simulink model "Two_Zone_MVDC_Ideal_ACDC"  (R2020b)
settings: Solver=FixedStepDiscrete  StartTime=0.0  StopTime=50  FixedStep=TsELEC  RelTol=1e-3  EnableMultiTasking=on
InitFcn:
  | TsELEC = 5e-4;
  | Ts = 5e-4;
undefined symbols (not defined in the file): DiscIntNeverNeededParam, droop1, droop2, GABDA, GABDB, GBBDA, GBBDB, GPMMA, GPPMB, GPPMC, SADA, SADB, SADC, SADD, SBDA, SBDB, SBDC, SCDA, SCDB, SCDC, SCDD, SDDA, SDDB, SDDC, SDDD, SDDE
libraries: fl_lib x66, nesl_utility x49, ee_lib x30, simulink x1
(part 1 of 2)
CloseFcn:
  | load initParams
settings Model: SimulationMode=accelerator  Creator=gdudgeon  LastModifiedBy=gdudgeon
settings SolverCC: ConcurrentTasks=on  AutoInsertRateTranBlk=on
settings DataIOCC: SaveFormat=StructureWithTime  SaveOutput=off  DSMLogging=off  SaveTime=off  ReturnWorkspaceOutputs=off
settings OptimizationCC: BlockReduction=off  OptimizeBlockIOStorage=off  BufferReuse=off  GlobalBufferReuse=off  ExpressionFolding=off  LocalBlockOutputs=off  OptimizeDataStoreBuffers=off  BusAssignmentInplaceUpdate=off
settings ModelReferenceCC: ModelReferenceNumInstancesAllowed=Single  ModelReferenceMinAlgLoopOccurrences=on
settings SFSimCC: CustomCodeUndefinedFunction=UseInterfaceOnly
settings RTWCC: TLCOptions=-axPCMaxOverloads=3000  RTWCompilerOptimization=on
settings GRTTargetCC: TargetLangStandard=C89/C90 (ANSI)

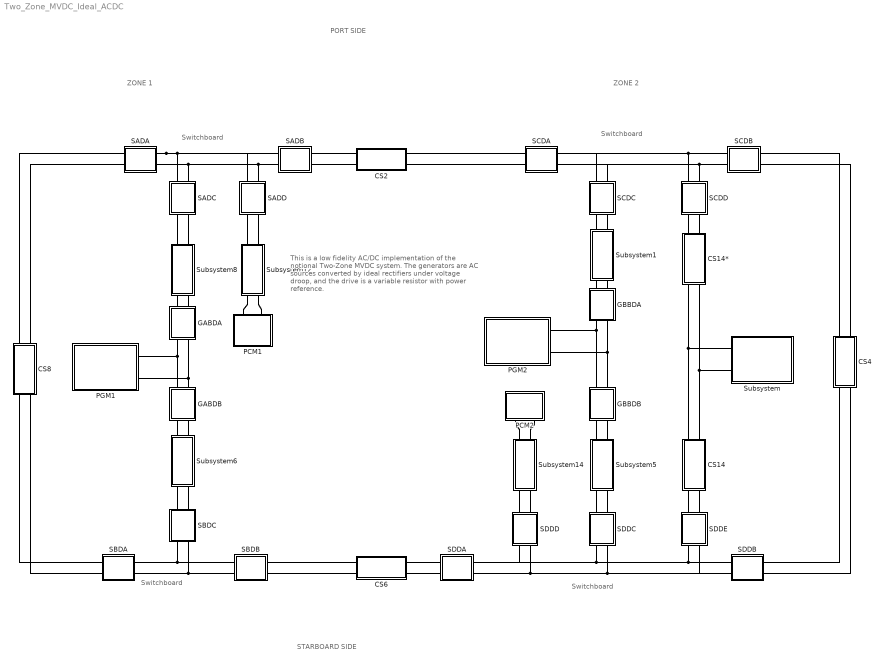
== system Two_Zone_MVDC_Ideal_ACDC ==
  note: This is a low fidelity
      | AC/DC implementation of the notional
      | Two-Zone MVDC system.
      | The generators are AC sources converted by ideal rectifiers under voltage droop, and the drive is a variable resistor with power reference.
  note: PORT SIDE
  note: Switchboard
  note: ZONE 1
  note: ZONE 2
  note: Switchboard
  note: Switchboard
  note: Switchboard
  note: STARBOARD SIDE
  CS14 : Subsystem
      mask Display: disp('CS14')
  CS14* : Subsystem
      mask Display: disp('CS14*')
  CS2 : Subsystem
      mask Display: disp('CS2')
  CS4 : Subsystem
      mask Display: disp('CS4')
  CS6 : Subsystem
      mask Display: disp('CS6')
  CS8 : Subsystem
      mask Display: disp('CS8')
  GABDA : Subsystem  mask{status=GABDA}
      mask prompts: status "Initial Status"
      mask init:
      | if ~status
      |     
      |     set(gcbh,'BackgroundColor','green')
      |     
      | elseif status
      |     
      |     set(gcbh,'BackgroundColor','red')
      |     
      | end
  GABDB : Subsystem  mask{status=GABDB}
      mask prompts: status "Initial Status"
      mask init:
      | if ~status
      |     
      |     set(gcbh,'BackgroundColor','green')
      |     
      | elseif status
      |     
      |     set(gcbh,'BackgroundColor','red')
      |     
      | end
  GBBDA : Subsystem  mask{status=GBBDA}
      mask prompts: status "Initial Status"
      mask init:
      | if ~status
      |     
      |     set(gcbh,'BackgroundColor','green')
      |     
      | elseif status
      |     
      |     set(gcbh,'BackgroundColor','red')
      |     
      | end
  GBBDB : Subsystem  mask{status=GBBDB}
      mask prompts: status "Initial Status"
      mask init:
      | if ~status
      |     
      |     set(gcbh,'BackgroundColor','green')
      |     
      | elseif status
      |     
      |     set(gcbh,'BackgroundColor','red')
      |     
      | end
  PCM1 : Subsystem
      mask Display: disp('PCM1')
  PCM2 : Subsystem
      mask Display: disp('PCM2')
  PGM1 : Subsystem
      mask Display: disp('PGM1')
  PGM2 : Subsystem
      mask Display: disp('PGM2')
  SADA : Subsystem  mask{status=SADA}
      mask prompts: status "Initial Status"
      mask init:
      | if ~status
      |     
      |     set(gcbh,'BackgroundColor','green')
      |     
      | elseif status
      |     
      |     set(gcbh,'BackgroundColor','red')
      |     
      | end
  SADB : Subsystem  mask{status=SADB}
      mask prompts: status "Initial Status"
      mask init:
      | if ~status
      |     
      |     set(gcbh,'BackgroundColor','green')
      |     
      | elseif status
      |     
      |     set(gcbh,'BackgroundColor','red')
      |     
      | end
  SADC : Subsystem  mask{status=SADC}
      mask prompts: status "Initial Status"
      mask init:
      | if ~status
      |     
      |     set(gcbh,'BackgroundColor','green')
      |     
      | elseif status
      |     
      |     set(gcbh,'BackgroundColor','red')
      |     
      | end
  SADD : Subsystem  mask{status=SADD}
      mask prompts: status "Initial Status"
      mask init:
      | if ~status
      |     
      |     set(gcbh,'BackgroundColor','green')
      |     
      | elseif status
      |     
      |     set(gcbh,'BackgroundColor','red')
      |     
      | end
  SBDA : Subsystem  mask{status=SBDA}
      mask prompts: status "Initial Status"
      mask init:
      | if ~status
      |     
      |     set(gcbh,'BackgroundColor','green')
      |     
      | elseif status
      |     
      |     set(gcbh,'BackgroundColor','red')
      |     
      | end
  SBDB : Subsystem  mask{status=SBDB}
      mask prompts: status "Initial Status"
      mask init:
      | if ~status
      |     
      |     set(gcbh,'BackgroundColor','green')
      |     
      | elseif status
      |     
      |     set(gcbh,'BackgroundColor','red')
      |     
      | end
  SBDC : Subsystem  mask{status=SBDC}
      mask prompts: status "Initial Status"
      mask init:
      | if ~status
      |     
      |     set(gcbh,'BackgroundColor','green')
      |     
      | elseif status
      |     
      |     set(gcbh,'BackgroundColor','red')
      |     
      | end
  SCDA : Subsystem  mask{status=SCDA}
      mask prompts: status "Initial Status"
      mask init:
      | if ~status
      |     
      |     set(gcbh,'BackgroundColor','green')
      |     
      | elseif status
      |     
      |     set(gcbh,'BackgroundColor','red')
      |     
      | end
  SCDB : Subsystem  mask{status=SCDB}
      mask prompts: status "Initial Status"
      mask init:
      | if ~status
      |     
      |     set(gcbh,'BackgroundColor','green')
      |     
      | elseif status
      |     
      |     set(gcbh,'BackgroundColor','red')
      |     
      | end
  SCDC : Subsystem  mask{status=SCDC}
      mask prompts: status "Initial Status"
      mask init:
      | if ~status
      |     
      |     set(gcbh,'BackgroundColor','green')
      |     
      | elseif status
      |     
      |     set(gcbh,'BackgroundColor','red')
      |     
      | end
  SCDD : Subsystem  mask{status=SCDD}
      mask prompts: status "Initial Status"
      mask init:
      | if ~status
      |     
      |     set(gcbh,'BackgroundColor','green')
      |     
      | elseif status
      |     
      |     set(gcbh,'BackgroundColor','red')
      |     
      | end
  SDDA : Subsystem  mask{status=SDDA}
      mask prompts: status "Initial Status"
      mask init:
      | if ~status
      |     
      |     set(gcbh,'BackgroundColor','green')
      |     
      | elseif status
      |     
      |     set(gcbh,'BackgroundColor','red')
      |     
      | end
  SDDB : Subsystem  mask{status=SDDB}
      mask prompts: status "Initial Status"
      mask init:
      | if ~status
      |     
      |     set(gcbh,'BackgroundColor','green')
      |     
      | elseif status
      |     
      |     set(gcbh,'BackgroundColor','red')
      |     
      | end
  SDDC : Subsystem  mask{status=SDDC}
      mask prompts: status "Initial Status"
      mask init:
      | if ~status
      |     
      |     set(gcbh,'BackgroundColor','green')
      |     
      | elseif status
      |     
      |     set(gcbh,'BackgroundColor','red')
      |     
      | end
  SDDD : Subsystem  mask{status=SDDD}
      mask prompts: status "Initial Status"
      mask init:
      | if ~status
      |     
      |     set(gcbh,'BackgroundColor','green')
      |     
      | elseif status
      |     
      |     set(gcbh,'BackgroundColor','red')
      |     
      | end
  SDDE : Subsystem  mask{status=SDDE}
      mask prompts: status "Initial Status"
      mask init:
      | if ~status
      |     
      |     set(gcbh,'BackgroundColor','green')
      |     
      | elseif status
      |     
      |     set(gcbh,'BackgroundColor','red')
      |     
      | end
  Subsystem : Subsystem
      mask Display: disp('PMM')
  Subsystem1 : Subsystem
      mask Display: disp('CS11*')
  Subsystem12 : Subsystem
      mask Display: disp('CS21')
  Subsystem14 : Subsystem
      mask Display: disp('CS22')
  Subsystem5 : Subsystem
      mask Display: disp('CS11')
  Subsystem6 : Subsystem
      mask Display: disp('CS9*')
  Subsystem8 : Subsystem
      mask Display: disp('CS9')
  connections:
  SADA/RConn2 -- SADC/LConn2 -- SADD/LConn2 -- SADB/LConn2
  SBDC/RConn2 -- SBDB/LConn2 -- SBDA/RConn2
  PGM1/RConn2 -- GABDB/LConn2 -- GABDA/RConn2
  PGM1/RConn1 -- GABDB/LConn1 -- GABDA/RConn1
  SADA/RConn1 -- SADD/LConn1 -- SADB/LConn1 -- SADC/LConn1
  SBDC/RConn1 -- SBDB/LConn1 -- SBDA/RConn1
  SCDA/LConn2 -- CS2/LConn2
  SADB/RConn1 -- CS2/RConn1
  Subsystem12/LConn1 -- SADD/RConn1
  SBDA/LConn2 -- CS8/RConn2
  SBDC/LConn1 -- Subsystem6/RConn1
  Subsystem12/RConn1 -- PCM1/LConn1
  SBDB/RConn1 -- CS6/RConn1
  SBDC/LConn2 -- Subsystem6/RConn2
  CS8/LConn1 -- SADA/LConn1
  Subsystem12/RConn2 -- PCM1/LConn2
  Subsystem12/LConn2 -- SADD/RConn2
  SADC/RConn1 -- Subsystem8/LConn1
  SBDB/RConn2 -- CS6/RConn2
  SADB/RConn2 -- CS2/RConn2
  CS8/LConn2 -- SADA/LConn2
  SBDA/LConn1 -- CS8/RConn1
  SADC/RConn2 -- Subsystem8/LConn2
  GBBDA/RConn1 -- GBBDB/LConn1 -- PGM2/RConn1
  SDDC/RConn2 -- SDDB/LConn2 -- SDDE/RConn2 -- SDDA/RConn2 -- SDDD/RConn2
  SCDC/LConn2 -- SCDA/RConn2 -- SCDD/LConn2 -- SCDB/LConn2
  SDDC/RConn1 -- SDDA/RConn1 -- SDDD/RConn1 -- SDDB/LConn1 -- SDDE/RConn1
  SCDC/LConn1 -- SCDA/RConn1 -- SCDD/LConn1 -- SCDB/LConn1
  GBBDA/RConn2 -- GBBDB/LConn2 -- PGM2/RConn2
  SCDC/RConn2 -- Subsystem1/LConn2
  SCDB/RConn1 -- CS4/LConn1
  SDDB/RConn1 -- CS4/RConn1
  SDDC/LConn2 -- Subsystem5/RConn2
  SDDB/RConn2 -- CS4/RConn2
  SCDB/RConn2 -- CS4/LConn2
  SDDC/LConn1 -- Subsystem5/RConn1
  SCDC/RConn1 -- Subsystem1/LConn1
  CS2/LConn1 -- SCDA/LConn1
  CS6/LConn1 -- SDDA/LConn1
  CS6/LConn2 -- SDDA/LConn2
  GBBDA/LConn1 -- Subsystem1/RConn1
  GBBDA/LConn2 -- Subsystem1/RConn2
  GBBDB/RConn1 -- Subsystem5/LConn1
  GBBDB/RConn2 -- Subsystem5/LConn2
  GABDA/LConn1 -- Subsystem8/RConn1
  GABDA/LConn2 -- Subsystem8/RConn2
  GABDB/RConn1 -- Subsystem6/LConn1
  GABDB/RConn2 -- Subsystem6/LConn2
  Subsystem14/LConn1 -- PCM2/LConn1
  Subsystem14/LConn2 -- PCM2/LConn2
  Subsystem14/RConn1 -- SDDD/LConn1
  Subsystem14/RConn2 -- SDDD/LConn2
  CS14*/LConn2 -- SCDD/RConn2
  CS14*/LConn1 -- SCDD/RConn1
  CS14/RConn1 -- SDDE/LConn1
  CS14/RConn2 -- SDDE/LConn2
  CS14/LConn1 -- Subsystem/LConn1 -- CS14*/RConn1
  CS14*/RConn2 -- Subsystem/LConn2 -- CS14/LConn2

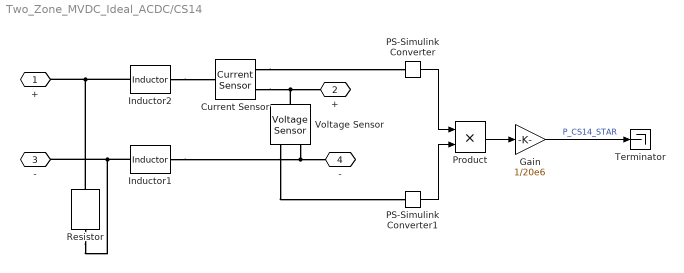
== system Two_Zone_MVDC_Ideal_ACDC/CS14 ==
  Current Sensor : fl_lib/Electrical/Electrical Sensors/Current Sensor
  Gain : Gain  Gain=1/20e6
  Inductor1 : fl_lib/Electrical/Electrical Elements/Inductor  l=5.32e-6 H  r=0.32e-3 Ohm  g=0 1/Ohm  i_specify=off  i_priority=None  i=0 A  i_nominal_specify=off  i_nominal_unit=A  i_nominal_value=1  v_specify=off  v_priority=None  v=0 V  v_nominal_specify=off  v_nominal_unit=V  v_nominal_value=1  i_L_specify=off  i_L_priority=High  i_L=0 A  i_L_nominal_specify=off  i_L_nominal_unit=A  i_L_nominal_value=1
  Inductor2 : fl_lib/Electrical/Electrical Elements/Inductor  l=5.32e-6 H  r=0.32e-3 Ohm  g=0 1/Ohm  i_specify=off  i_priority=None  i=0 A  i_nominal_specify=off  i_nominal_unit=A  i_nominal_value=1  v_specify=off  v_priority=None  v=0 V  v_nominal_specify=off  v_nominal_unit=V  v_nominal_value=1  i_L_specify=off  i_L_priority=High  i_L=0 A  i_L_nominal_specify=off  i_L_nominal_unit=A  i_L_nominal_value=1
  PS-Simulink Converter : nesl_utility/PS-Simulink Converter  PhysicalDomain=network_engine_domain  SubClassName=ps_output  LeftPortType=input  RightPortType=output  PseudoPeriodic=off  Frequencies=[]  Unit=inherit  AffineConversion=off
  PS-Simulink Converter1 : nesl_utility/PS-Simulink Converter  PhysicalDomain=network_engine_domain  SubClassName=ps_output  LeftPortType=input  RightPortType=output  PseudoPeriodic=off  Frequencies=[]  Unit=inherit  AffineConversion=off
  Product : Product
  Resistor : fl_lib/Electrical/Electrical Elements/Resistor  R=1e4 Ohm  i_specify=off  i_priority=None  i=0 A  i_nominal_specify=off  i_nominal_unit=A  i_nominal_value=1  v_specify=off  v_priority=None  v=0 V  v_nominal_specify=off  v_nominal_unit=V  v_nominal_value=1
  Terminator : Terminator
  Voltage Sensor : fl_lib/Electrical/Electrical Sensors/Voltage Sensor
  "+ " : PMIOPort  Side=Left
  + : PMIOPort  Port=2  Side=Right
  - : PMIOPort  Port=3  Side=Left
  "- " : PMIOPort  Port=4  Side=Right
  wires:
  PS-Simulink Converter/1 -> Product/1
  PS-Simulink Converter1/1 -> Product/2
  Product/1 -> Gain/1
  Gain/1 -> Terminator/1  "P_CS14_STAR"
  connections:
  Inductor1/LConn1 -- Resistor/RConn1 -- -/RConn1
  Inductor2/LConn1 -- Resistor/LConn1 -- "+ "/RConn1
  Inductor1/RConn1 -- Voltage Sensor/RConn2 -- "- "/RConn1
  Inductor2/RConn1 -- Current Sensor/LConn1
  Current Sensor/RConn2 -- Voltage Sensor/LConn1 -- +/RConn1
  Current Sensor/RConn1 -- PS-Simulink Converter/LConn1
  Voltage Sensor/RConn1 -- PS-Simulink Converter1/LConn1

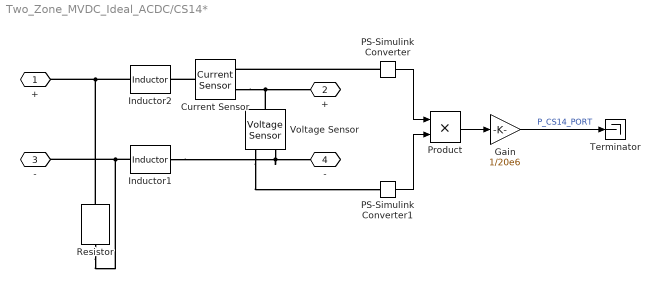
== system Two_Zone_MVDC_Ideal_ACDC/CS14* ==
  Current Sensor : fl_lib/Electrical/Electrical Sensors/Current Sensor
  Gain : Gain  Gain=1/20e6
  Inductor1 : fl_lib/Electrical/Electrical Elements/Inductor  l=5.32e-6 H  r=0.32e-3 Ohm  g=0 1/Ohm  i_specify=off  i_priority=None  i=0 A  i_nominal_specify=off  i_nominal_unit=A  i_nominal_value=1  v_specify=off  v_priority=None  v=0 V  v_nominal_specify=off  v_nominal_unit=V  v_nominal_value=1  i_L_specify=off  i_L_priority=High  i_L=0 A  i_L_nominal_specify=off  i_L_nominal_unit=A  i_L_nominal_value=1
  Inductor2 : fl_lib/Electrical/Electrical Elements/Inductor  l=5.32e-6 H  r=0.32e-3 Ohm  g=0 1/Ohm  i_specify=off  i_priority=None  i=0 A  i_nominal_specify=off  i_nominal_unit=A  i_nominal_value=1  v_specify=off  v_priority=None  v=0 V  v_nominal_specify=off  v_nominal_unit=V  v_nominal_value=1  i_L_specify=off  i_L_priority=High  i_L=0 A  i_L_nominal_specify=off  i_L_nominal_unit=A  i_L_nominal_value=1
  PS-Simulink Converter : nesl_utility/PS-Simulink Converter  PhysicalDomain=network_engine_domain  SubClassName=ps_output  LeftPortType=input  RightPortType=output  PseudoPeriodic=off  Frequencies=[]  Unit=inherit  AffineConversion=off
  PS-Simulink Converter1 : nesl_utility/PS-Simulink Converter  PhysicalDomain=network_engine_domain  SubClassName=ps_output  LeftPortType=input  RightPortType=output  PseudoPeriodic=off  Frequencies=[]  Unit=inherit  AffineConversion=off
  Product : Product
  Resistor : fl_lib/Electrical/Electrical Elements/Resistor  R=1e4 Ohm  i_specify=off  i_priority=None  i=0 A  i_nominal_specify=off  i_nominal_unit=A  i_nominal_value=1  v_specify=off  v_priority=None  v=0 V  v_nominal_specify=off  v_nominal_unit=V  v_nominal_value=1
  Terminator : Terminator
  Voltage Sensor : fl_lib/Electrical/Electrical Sensors/Voltage Sensor
  "+ " : PMIOPort  Side=Left
  + : PMIOPort  Port=2  Side=Right
  - : PMIOPort  Port=3  Side=Left
  "- " : PMIOPort  Port=4  Side=Right
  wires:
  PS-Simulink Converter/1 -> Product/1
  PS-Simulink Converter1/1 -> Product/2
  Product/1 -> Gain/1
  Gain/1 -> Terminator/1  "P_CS14_PORT"
  connections:
  Inductor1/RConn1 -- Voltage Sensor/RConn2 -- "- "/RConn1
  Inductor2/LConn1 -- Resistor/LConn1 -- "+ "/RConn1
  Inductor1/LConn1 -- Resistor/RConn1 -- -/RConn1
  Current Sensor/LConn1 -- Inductor2/RConn1
  Current Sensor/RConn2 -- Voltage Sensor/LConn1 -- +/RConn1
  PS-Simulink Converter/LConn1 -- Current Sensor/RConn1
  Voltage Sensor/RConn1 -- PS-Simulink Converter1/LConn1

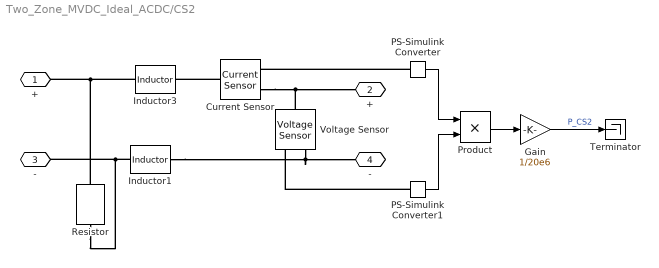
== system Two_Zone_MVDC_Ideal_ACDC/CS2 ==
  Current Sensor : fl_lib/Electrical/Electrical Sensors/Current Sensor
  Gain : Gain  Gain=1/20e6
  Inductor1 : fl_lib/Electrical/Electrical Elements/Inductor  l=3.47e-6 H  r=0.21e-3 Ohm  g=0 1/Ohm  i_specify=off  i_priority=None  i=0 A  i_nominal_specify=off  i_nominal_unit=A  i_nominal_value=1  v_specify=off  v_priority=None  v=0 V  v_nominal_specify=off  v_nominal_unit=V  v_nominal_value=1  i_L_specify=off  i_L_priority=High  i_L=0 A  i_L_nominal_specify=off  i_L_nominal_unit=A  i_L_nominal_value=1
  Inductor3 : fl_lib/Electrical/Electrical Elements/Inductor  l=3.47e-6 H  r=0.21e-3 Ohm  g=0 1/Ohm  i_specify=off  i_priority=None  i=0 A  i_nominal_specify=off  i_nominal_unit=A  i_nominal_value=1  v_specify=off  v_priority=None  v=0 V  v_nominal_specify=off  v_nominal_unit=V  v_nominal_value=1  i_L_specify=off  i_L_priority=High  i_L=0 A  i_L_nominal_specify=off  i_L_nominal_unit=A  i_L_nominal_value=1
  PS-Simulink Converter : nesl_utility/PS-Simulink Converter  PhysicalDomain=network_engine_domain  SubClassName=ps_output  LeftPortType=input  RightPortType=output  PseudoPeriodic=off  Frequencies=[]  Unit=inherit  AffineConversion=off
  PS-Simulink Converter1 : nesl_utility/PS-Simulink Converter  PhysicalDomain=network_engine_domain  SubClassName=ps_output  LeftPortType=input  RightPortType=output  PseudoPeriodic=off  Frequencies=[]  Unit=inherit  AffineConversion=off
  Product : Product
  Resistor : fl_lib/Electrical/Electrical Elements/Resistor  R=1e4 Ohm  i_specify=off  i_priority=None  i=0 A  i_nominal_specify=off  i_nominal_unit=A  i_nominal_value=1  v_specify=off  v_priority=None  v=0 V  v_nominal_specify=off  v_nominal_unit=V  v_nominal_value=1
  Terminator : Terminator
  Voltage Sensor : fl_lib/Electrical/Electrical Sensors/Voltage Sensor
  "+ " : PMIOPort  Side=Left
  + : PMIOPort  Port=2  Side=Right
  - : PMIOPort  Port=3  Side=Left
  "- " : PMIOPort  Port=4  Side=Right
  wires:
  PS-Simulink Converter/1 -> Product/1
  PS-Simulink Converter1/1 -> Product/2
  Product/1 -> Gain/1
  Gain/1 -> Terminator/1  "P_CS2"
  connections:
  Inductor3/LConn1 -- Resistor/LConn1 -- "+ "/RConn1
  Inductor1/LConn1 -- Resistor/RConn1 -- -/RConn1
  Inductor1/RConn1 -- Voltage Sensor/RConn2 -- "- "/RConn1
  Current Sensor/LConn1 -- Inductor3/RConn1
  Current Sensor/RConn2 -- Voltage Sensor/LConn1 -- +/RConn1
  PS-Simulink Converter/LConn1 -- Current Sensor/RConn1
  PS-Simulink Converter1/LConn1 -- Voltage Sensor/RConn1

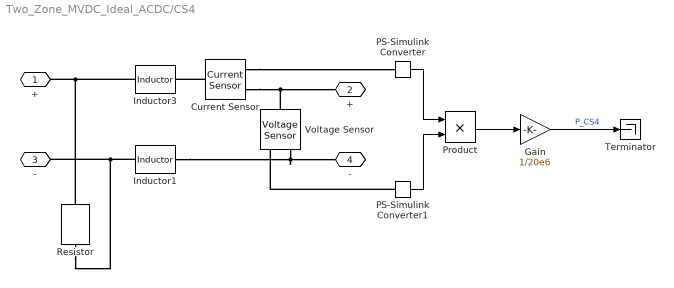
== system Two_Zone_MVDC_Ideal_ACDC/CS4 ==
  Current Sensor : fl_lib/Electrical/Electrical Sensors/Current Sensor
  Gain : Gain  Gain=1/20e6
  Inductor1 : fl_lib/Electrical/Electrical Elements/Inductor  l=5e-6 H  r=0.2e-3 Ohm  g=0 1/Ohm  i_specify=off  i_priority=None  i=0 A  i_nominal_specify=off  i_nominal_unit=A  i_nominal_value=1  v_specify=off  v_priority=None  v=0 V  v_nominal_specify=off  v_nominal_unit=V  v_nominal_value=1  i_L_specify=off  i_L_priority=High  i_L=0 A  i_L_nominal_specify=off  i_L_nominal_unit=A  i_L_nominal_value=1
  Inductor3 : fl_lib/Electrical/Electrical Elements/Inductor  l=5e-6 H  r=0.2e-3 Ohm  g=0 1/Ohm  i_specify=off  i_priority=None  i=0 A  i_nominal_specify=off  i_nominal_unit=A  i_nominal_value=1  v_specify=off  v_priority=None  v=0 V  v_nominal_specify=off  v_nominal_unit=V  v_nominal_value=1  i_L_specify=off  i_L_priority=High  i_L=0 A  i_L_nominal_specify=off  i_L_nominal_unit=A  i_L_nominal_value=1
  PS-Simulink Converter : nesl_utility/PS-Simulink Converter  PhysicalDomain=network_engine_domain  SubClassName=ps_output  LeftPortType=input  RightPortType=output  PseudoPeriodic=off  Frequencies=[]  Unit=inherit  AffineConversion=off
  PS-Simulink Converter1 : nesl_utility/PS-Simulink Converter  PhysicalDomain=network_engine_domain  SubClassName=ps_output  LeftPortType=input  RightPortType=output  PseudoPeriodic=off  Frequencies=[]  Unit=inherit  AffineConversion=off
  Product : Product
  Resistor : fl_lib/Electrical/Electrical Elements/Resistor  R=1e4 Ohm  i_specify=off  i_priority=None  i=0 A  i_nominal_specify=off  i_nominal_unit=A  i_nominal_value=1  v_specify=off  v_priority=None  v=0 V  v_nominal_specify=off  v_nominal_unit=V  v_nominal_value=1
  Terminator : Terminator
  Voltage Sensor : fl_lib/Electrical/Electrical Sensors/Voltage Sensor
  "+ " : PMIOPort  Side=Left
  + : PMIOPort  Port=2  Side=Right
  - : PMIOPort  Port=3  Side=Left
  "- " : PMIOPort  Port=4  Side=Right
  wires:
  Product/1 -> Gain/1
  PS-Simulink Converter/1 -> Product/1
  PS-Simulink Converter1/1 -> Product/2
  Gain/1 -> Terminator/1  "P_CS4"
  connections:
  Inductor3/LConn1 -- Resistor/LConn1 -- "+ "/RConn1
  Inductor1/LConn1 -- Resistor/RConn1 -- -/RConn1
  Current Sensor/LConn1 -- Inductor3/RConn1
  Current Sensor/RConn2 -- Voltage Sensor/LConn1 -- +/RConn1
  Inductor1/RConn1 -- Voltage Sensor/RConn2 -- "- "/RConn1
  Current Sensor/RConn1 -- PS-Simulink Converter/LConn1
  PS-Simulink Converter1/LConn1 -- Voltage Sensor/RConn1

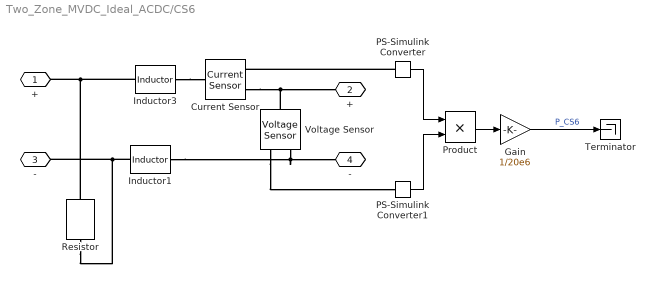
== system Two_Zone_MVDC_Ideal_ACDC/CS6 ==
  Current Sensor : fl_lib/Electrical/Electrical Sensors/Current Sensor
  Gain : Gain  Gain=1/20e6
  Inductor1 : fl_lib/Electrical/Electrical Elements/Inductor  l=3.47e-6 H  r=0.21e-3 Ohm  g=0 1/Ohm  i_specify=off  i_priority=None  i=0 A  i_nominal_specify=off  i_nominal_unit=A  i_nominal_value=1  v_specify=off  v_priority=None  v=0 V  v_nominal_specify=off  v_nominal_unit=V  v_nominal_value=1  i_L_specify=off  i_L_priority=High  i_L=0 A  i_L_nominal_specify=off  i_L_nominal_unit=A  i_L_nominal_value=1
  Inductor3 : fl_lib/Electrical/Electrical Elements/Inductor  l=3.47e-6 H  r=0.21e-3 Ohm  g=0 1/Ohm  i_specify=off  i_priority=None  i=0 A  i_nominal_specify=off  i_nominal_unit=A  i_nominal_value=1  v_specify=off  v_priority=None  v=0 V  v_nominal_specify=off  v_nominal_unit=V  v_nominal_value=1  i_L_specify=off  i_L_priority=High  i_L=0 A  i_L_nominal_specify=off  i_L_nominal_unit=A  i_L_nominal_value=1
  PS-Simulink Converter : nesl_utility/PS-Simulink Converter  PhysicalDomain=network_engine_domain  SubClassName=ps_output  LeftPortType=input  RightPortType=output  PseudoPeriodic=off  Frequencies=[]  Unit=inherit  AffineConversion=off
  PS-Simulink Converter1 : nesl_utility/PS-Simulink Converter  PhysicalDomain=network_engine_domain  SubClassName=ps_output  LeftPortType=input  RightPortType=output  PseudoPeriodic=off  Frequencies=[]  Unit=inherit  AffineConversion=off
  Product : Product
  Resistor : fl_lib/Electrical/Electrical Elements/Resistor  R=1e4 Ohm  i_specify=off  i_priority=None  i=0 A  i_nominal_specify=off  i_nominal_unit=A  i_nominal_value=1  v_specify=off  v_priority=None  v=0 V  v_nominal_specify=off  v_nominal_unit=V  v_nominal_value=1
  Terminator : Terminator
  Voltage Sensor : fl_lib/Electrical/Electrical Sensors/Voltage Sensor
  "+ " : PMIOPort  Side=Left
  + : PMIOPort  Port=2  Side=Right
  - : PMIOPort  Port=3  Side=Left
  "- " : PMIOPort  Port=4  Side=Right
  wires:
  Product/1 -> Gain/1
  PS-Simulink Converter/1 -> Product/1
  PS-Simulink Converter1/1 -> Product/2
  Gain/1 -> Terminator/1  "P_CS6"
  connections:
  Inductor1/LConn1 -- Resistor/RConn1 -- -/RConn1
  Inductor3/LConn1 -- Resistor/LConn1 -- "+ "/RConn1
  Inductor3/RConn1 -- Current Sensor/LConn1
  Current Sensor/RConn2 -- Voltage Sensor/LConn1 -- +/RConn1
  Inductor1/RConn1 -- Voltage Sensor/RConn2 -- "- "/RConn1
  Voltage Sensor/RConn1 -- PS-Simulink Converter1/LConn1
  PS-Simulink Converter/LConn1 -- Current Sensor/RConn1

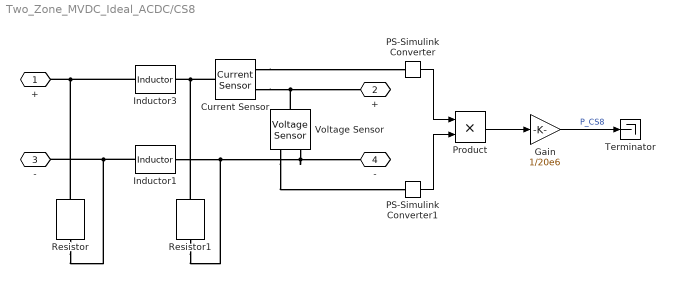
== system Two_Zone_MVDC_Ideal_ACDC/CS8 ==
  Current Sensor : fl_lib/Electrical/Electrical Sensors/Current Sensor
  Gain : Gain  Gain=1/20e6
  Inductor1 : fl_lib/Electrical/Electrical Elements/Inductor  l=5e-6 H  r=0.2e-3 Ohm  g=0 1/Ohm  i_specify=off  i_priority=None  i=0 A  i_nominal_specify=off  i_nominal_unit=A  i_nominal_value=1  v_specify=off  v_priority=None  v=0 V  v_nominal_specify=off  v_nominal_unit=V  v_nominal_value=1  i_L_specify=off  i_L_priority=High  i_L=0 A  i_L_nominal_specify=off  i_L_nominal_unit=A  i_L_nominal_value=1
  Inductor3 : fl_lib/Electrical/Electrical Elements/Inductor  l=5e-6 H  r=0.2e-3 Ohm  g=0 1/Ohm  i_specify=off  i_priority=None  i=0 A  i_nominal_specify=off  i_nominal_unit=A  i_nominal_value=1  v_specify=off  v_priority=None  v=0 V  v_nominal_specify=off  v_nominal_unit=V  v_nominal_value=1  i_L_specify=off  i_L_priority=High  i_L=0 A  i_L_nominal_specify=off  i_L_nominal_unit=A  i_L_nominal_value=1
  PS-Simulink Converter : nesl_utility/PS-Simulink Converter  PhysicalDomain=network_engine_domain  SubClassName=ps_output  LeftPortType=input  RightPortType=output  PseudoPeriodic=off  Frequencies=[]  Unit=inherit  AffineConversion=off
  PS-Simulink Converter1 : nesl_utility/PS-Simulink Converter  PhysicalDomain=network_engine_domain  SubClassName=ps_output  LeftPortType=input  RightPortType=output  PseudoPeriodic=off  Frequencies=[]  Unit=inherit  AffineConversion=off
  Product : Product
  Resistor : fl_lib/Electrical/Electrical Elements/Resistor  R=1e4 Ohm  i_specify=off  i_priority=None  i=0 A  i_nominal_specify=off  i_nominal_unit=A  i_nominal_value=1  v_specify=off  v_priority=None  v=0 V  v_nominal_specify=off  v_nominal_unit=V  v_nominal_value=1
  Resistor1 : fl_lib/Electrical/Electrical Elements/Resistor  R=1e4 Ohm  i_specify=off  i_priority=None  i=0 A  i_nominal_specify=off  i_nominal_unit=A  i_nominal_value=1  v_specify=off  v_priority=None  v=0 V  v_nominal_specify=off  v_nominal_unit=V  v_nominal_value=1
  Terminator : Terminator
  Voltage Sensor : fl_lib/Electrical/Electrical Sensors/Voltage Sensor
  "+ " : PMIOPort  Side=Left
  + : PMIOPort  Port=2  Side=Right
  - : PMIOPort  Port=3  Side=Left
  "- " : PMIOPort  Port=4  Side=Right
  wires:
  Product/1 -> Gain/1
  PS-Simulink Converter/1 -> Product/1
  PS-Simulink Converter1/1 -> Product/2
  Gain/1 -> Terminator/1  "P_CS8"
  connections:
  Inductor1/LConn1 -- Resistor/RConn1 -- -/RConn1
  Inductor3/LConn1 -- Resistor/LConn1 -- "+ "/RConn1
  Current Sensor/LConn1 -- Resistor1/LConn1 -- Inductor3/RConn1
  Current Sensor/RConn2 -- Voltage Sensor/LConn1 -- +/RConn1
  Inductor1/RConn1 -- Resistor1/RConn1 -- Voltage Sensor/RConn2 -- "- "/RConn1
  Voltage Sensor/RConn1 -- PS-Simulink Converter1/LConn1
  Current Sensor/RConn1 -- PS-Simulink Converter/LConn1

== system Two_Zone_MVDC_Ideal_ACDC/GABDA ==
  GABDA : ee_lib/Switches & Breakers/DPST Switch  R_closed=1e-4 Ohm  G_open=1e-6 S  Threshold=0.5 V  Width=0 V  model_dynamics=0  t_on=1e-3 s  t_off=1e-3 s  initial_vT=0 V
      settings: SourceProductBaseCode=PS  InternalSimscapePortConfiguration="{\"Bottom\":[],\"Left\":[{\"id\":\"vT\",\"label\":\"vT\",\"type\":\"input\"},{\"id\":\"p1\",\"label\":\"\",\"type\":\"foundation.electrical.electrical\"},{\"id\":\"p2\",\"label\":\"\",\"type\":\"foundation.electrical.electrical\"}],\"Right\":[{\"id\":\"n1\",\"label\":\"\",\"type\":\"foundation.electrical.electrical\"},{\"id\":\"n2\",\"label\":\"\",\"type\":\"foundation.electrical.electrical\"}],\"Top\":[]}"
  Simulink-PS Converter : nesl_utility/Simulink-PS Converter  PhysicalDomain=network_engine_domain  SubClassName=ps_input  LeftPortType=input  RightPortType=output  PseudoPeriodic=off  Frequencies=[]  NoiseDistribution=none  NoiseParameters=[]  Unit=1  AffineConversion=off  FilteringAndDerivatives=provide  SimscapeFilterOrder=1  InputFilterTimeConstant=0.001  UdotUserProvided=0
  "+ " : PMIOPort  Side=Right
  + : PMIOPort  Port=2  Side=Left
  "- " : PMIOPort  Port=3  Side=Right
  - : PMIOPort  Port=4  Side=Left
  wires:
  [GABDA] -> Simulink-PS Converter/1
  connections:
  GABDA/RConn1 -- "+ "/RConn1
  GABDA/LConn3 -- -/RConn1
  GABDA/RConn2 -- "- "/RConn1
  Simulink-PS Converter/RConn1 -- GABDA/LConn1
  GABDA/LConn2 -- +/RConn1

== system Two_Zone_MVDC_Ideal_ACDC/GABDB ==
  GABDB : ee_lib/Switches & Breakers/DPST Switch  R_closed=1e-4 Ohm  G_open=1e-6 S  Threshold=0.5 V  Width=0 V  model_dynamics=0  t_on=1e-3 s  t_off=1e-3 s  initial_vT=0 V
      settings: SourceProductBaseCode=PS  InternalSimscapePortConfiguration="{\"Bottom\":[],\"Left\":[{\"id\":\"vT\",\"label\":\"vT\",\"type\":\"input\"},{\"id\":\"p1\",\"label\":\"\",\"type\":\"foundation.electrical.electrical\"},{\"id\":\"p2\",\"label\":\"\",\"type\":\"foundation.electrical.electrical\"}],\"Right\":[{\"id\":\"n1\",\"label\":\"\",\"type\":\"foundation.electrical.electrical\"},{\"id\":\"n2\",\"label\":\"\",\"type\":\"foundation.electrical.electrical\"}],\"Top\":[]}"
  Simulink-PS Converter : nesl_utility/Simulink-PS Converter  PhysicalDomain=network_engine_domain  SubClassName=ps_input  LeftPortType=input  RightPortType=output  PseudoPeriodic=off  Frequencies=[]  NoiseDistribution=none  NoiseParameters=[]  Unit=1  AffineConversion=off  FilteringAndDerivatives=provide  SimscapeFilterOrder=1  InputFilterTimeConstant=0.001  UdotUserProvided=0
  "+ " : PMIOPort  Side=Right
  + : PMIOPort  Port=2  Side=Left
  "- " : PMIOPort  Port=3  Side=Right
  - : PMIOPort  Port=4  Side=Left
  wires:
  [GABDB] -> Simulink-PS Converter/1
  connections:
  GABDB/LConn2 -- +/RConn1
  Simulink-PS Converter/RConn1 -- GABDB/LConn1
  GABDB/RConn2 -- "- "/RConn1
  GABDB/LConn3 -- -/RConn1
  GABDB/RConn1 -- "+ "/RConn1

== system Two_Zone_MVDC_Ideal_ACDC/GBBDA ==
  GBBDA : ee_lib/Switches & Breakers/DPST Switch  R_closed=1e-4 Ohm  G_open=1e-6 S  Threshold=0.5 V  Width=0 V  model_dynamics=0  t_on=1e-3 s  t_off=1e-3 s  initial_vT=0 V
      settings: SourceProductBaseCode=PS  InternalSimscapePortConfiguration="{\"Bottom\":[],\"Left\":[{\"id\":\"vT\",\"label\":\"vT\",\"type\":\"input\"},{\"id\":\"p1\",\"label\":\"\",\"type\":\"foundation.electrical.electrical\"},{\"id\":\"p2\",\"label\":\"\",\"type\":\"foundation.electrical.electrical\"}],\"Right\":[{\"id\":\"n1\",\"label\":\"\",\"type\":\"foundation.electrical.electrical\"},{\"id\":\"n2\",\"label\":\"\",\"type\":\"foundation.electrical.electrical\"}],\"Top\":[]}"
  Simulink-PS Converter : nesl_utility/Simulink-PS Converter  PhysicalDomain=network_engine_domain  SubClassName=ps_input  LeftPortType=input  RightPortType=output  PseudoPeriodic=off  Frequencies=[]  NoiseDistribution=none  NoiseParameters=[]  Unit=1  AffineConversion=off  FilteringAndDerivatives=provide  SimscapeFilterOrder=1  InputFilterTimeConstant=0.001  UdotUserProvided=0
  "+ " : PMIOPort  Side=Right
  + : PMIOPort  Port=2  Side=Left
  "- " : PMIOPort  Port=3  Side=Right
  - : PMIOPort  Port=4  Side=Left
  wires:
  [GBBDA] -> Simulink-PS Converter/1
  connections:
  GBBDA/RConn1 -- "+ "/RConn1
  GBBDA/LConn3 -- -/RConn1
  GBBDA/RConn2 -- "- "/RConn1
  Simulink-PS Converter/RConn1 -- GBBDA/LConn1
  GBBDA/LConn2 -- +/RConn1

== system Two_Zone_MVDC_Ideal_ACDC/GBBDB ==
  GBBDB : ee_lib/Switches & Breakers/DPST Switch  R_closed=1e-4 Ohm  G_open=1e-6 S  Threshold=0.5 V  Width=0 V  model_dynamics=0  t_on=1e-3 s  t_off=1e-3 s  initial_vT=0 V
      settings: SourceProductBaseCode=PS  InternalSimscapePortConfiguration="{\"Bottom\":[],\"Left\":[{\"id\":\"vT\",\"label\":\"vT\",\"type\":\"input\"},{\"id\":\"p1\",\"label\":\"\",\"type\":\"foundation.electrical.electrical\"},{\"id\":\"p2\",\"label\":\"\",\"type\":\"foundation.electrical.electrical\"}],\"Right\":[{\"id\":\"n1\",\"label\":\"\",\"type\":\"foundation.electrical.electrical\"},{\"id\":\"n2\",\"label\":\"\",\"type\":\"foundation.electrical.electrical\"}],\"Top\":[]}"
  Simulink-PS Converter : nesl_utility/Simulink-PS Converter  PhysicalDomain=network_engine_domain  SubClassName=ps_input  LeftPortType=input  RightPortType=output  PseudoPeriodic=off  Frequencies=[]  NoiseDistribution=none  NoiseParameters=[]  Unit=1  AffineConversion=off  FilteringAndDerivatives=provide  SimscapeFilterOrder=1  InputFilterTimeConstant=0.001  UdotUserProvided=0
  "+ " : PMIOPort  Side=Right
  + : PMIOPort  Port=2  Side=Left
  "- " : PMIOPort  Port=3  Side=Right
  - : PMIOPort  Port=4  Side=Left
  wires:
  [GBBDB] -> Simulink-PS Converter/1
  connections:
  GBBDB/LConn2 -- +/RConn1
  Simulink-PS Converter/RConn1 -- GBBDB/LConn1
  GBBDB/RConn2 -- "- "/RConn1
  GBBDB/LConn3 -- -/RConn1
  GBBDB/RConn1 -- "+ "/RConn1

== system Two_Zone_MVDC_Ideal_ACDC/PCM1 ==
  Bus Creator : BusCreator  Inputs=3
  Current Sensor : fl_lib/Electrical/Electrical Sensors/Current Sensor
  PS-Simulink Converter : nesl_utility/PS-Simulink Converter  PhysicalDomain=network_engine_domain  SubClassName=ps_output  LeftPortType=input  RightPortType=output  PseudoPeriodic=off  Frequencies=[]  Unit=1  AffineConversion=off
  PS-Simulink Converter1 : nesl_utility/PS-Simulink Converter  PhysicalDomain=network_engine_domain  SubClassName=ps_output  LeftPortType=input  RightPortType=output  PseudoPeriodic=off  Frequencies=[]  Unit=1  AffineConversion=off
  Product : Product
  Resistor : fl_lib/Electrical/Electrical Elements/Resistor  R=100 Ohm  i_specify=off  i_priority=None  i=0 A  i_nominal_specify=off  i_nominal_unit=A  i_nominal_value=1  v_specify=off  v_priority=None  v=0 V  v_nominal_specify=off  v_nominal_unit=V  v_nominal_value=1
  Terminator : Terminator
  Voltage Sensor : fl_lib/Electrical/Electrical Sensors/Voltage Sensor
  + : PMIOPort  Side=Left
  - : PMIOPort  Port=2  Side=Left
  wires:
  Bus Creator/1 -> Terminator/1  "PCM1"
  Product/1 -> Bus Creator/3  "P"
  PS-Simulink Converter1/1 -> Bus Creator/2, Product/2  "V"
  PS-Simulink Converter/1 -> Bus Creator/1, Product/1  "I"
  connections:
  Current Sensor/LConn1 -- +/RConn1
  Voltage Sensor/RConn1 -- PS-Simulink Converter1/LConn1
  PS-Simulink Converter/LConn1 -- Current Sensor/RConn1
  Resistor/RConn1 -- -/RConn1 -- Voltage Sensor/RConn2
  Voltage Sensor/LConn1 -- Resistor/LConn1 -- Current Sensor/RConn2

== system Two_Zone_MVDC_Ideal_ACDC/PCM2 ==
  Bus Creator : BusCreator  Inputs=3
  Current Sensor : fl_lib/Electrical/Electrical Sensors/Current Sensor
  PS-Simulink Converter : nesl_utility/PS-Simulink Converter  PhysicalDomain=network_engine_domain  SubClassName=ps_output  LeftPortType=input  RightPortType=output  PseudoPeriodic=off  Frequencies=[]  Unit=1  AffineConversion=off
  PS-Simulink Converter1 : nesl_utility/PS-Simulink Converter  PhysicalDomain=network_engine_domain  SubClassName=ps_output  LeftPortType=input  RightPortType=output  PseudoPeriodic=off  Frequencies=[]  Unit=1  AffineConversion=off
  Product : Product
  Resistor : fl_lib/Electrical/Electrical Elements/Resistor  R=100 Ohm  i_specify=off  i_priority=None  i=0 A  i_nominal_specify=off  i_nominal_unit=A  i_nominal_value=1  v_specify=off  v_priority=None  v=0 V  v_nominal_specify=off  v_nominal_unit=V  v_nominal_value=1
  Terminator : Terminator
  Voltage Sensor : fl_lib/Electrical/Electrical Sensors/Voltage Sensor
  + : PMIOPort  Side=Left
  - : PMIOPort  Port=2  Side=Left
  wires:
  Bus Creator/1 -> Terminator/1  "PCM2"
  Product/1 -> Bus Creator/3  "P"
  PS-Simulink Converter1/1 -> Bus Creator/2, Product/2  "V"
  PS-Simulink Converter/1 -> Bus Creator/1, Product/1  "I"
  connections:
  +/RConn1 -- Current Sensor/LConn1
  Voltage Sensor/RConn1 -- PS-Simulink Converter1/LConn1
  PS-Simulink Converter/LConn1 -- Current Sensor/RConn1
  Resistor/RConn1 -- -/RConn1 -- Voltage Sensor/RConn2
  Voltage Sensor/LConn1 -- Resistor/LConn1 -- Current Sensor/RConn2

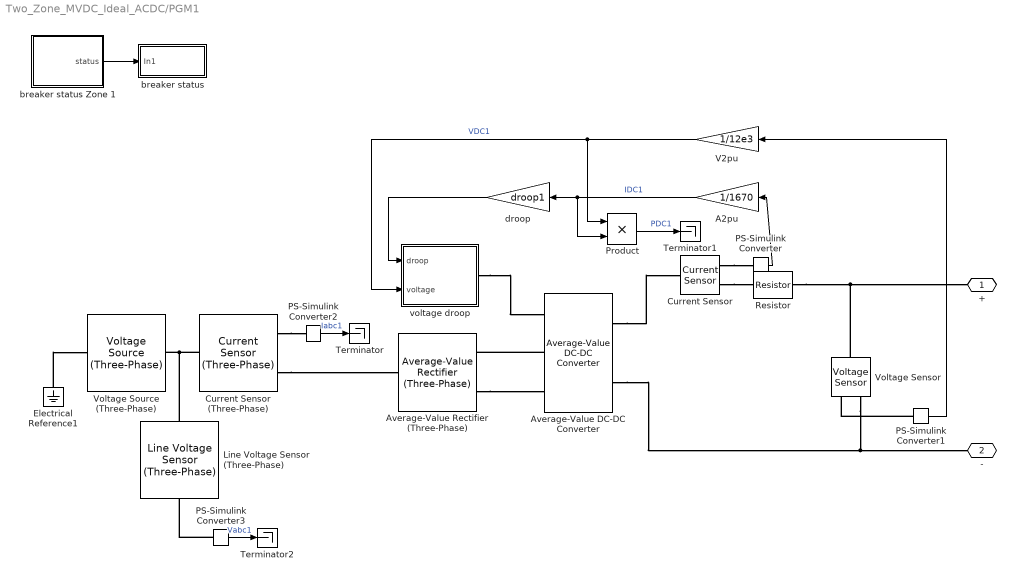
== system Two_Zone_MVDC_Ideal_ACDC/PGM1 ==
  A2pu : Gain  Gain=1/1670
  Average-Value Rectifier (Three-Phase) : ee_lib/Semiconductors & Converters/Converters/Average-Value Rectifier (Three-Phase)  VRated=12e3 V  Pfixed=1e4 W
      settings: SourceProductBaseCode=PS  InternalSimscapePortConfiguration="{\"Bottom\":[],\"Left\":[{\"id\":\"N\",\"label\":\"~\",\"type\":\"foundation.electrical.three_phase\"}],\"Right\":[{\"id\":\"p\",\"label\":\"+\",\"type\":\"foundation.electrical.electrical\"},{\"id\":\"n\",\"label\":\"-\",\"type\":\"foundation.electrical.electrical\"}],\"Top\":[]}"
  Average-Value DC-DC Converter : ee_lib/Semiconductors & Converters/Converters/Average-Value DC-DC Converter  control_option=ee.enum.converters.controlinput.dutycycle  converter_type=ee.enum.converters.dcdctype.buck  efficiency_option=ee.enum.converters.efficiency.constant  efficiency_fixed=100  i_vec=[0, 2, 5] A  efficiency_vec=[90, 95, 98]
      settings: SourceProductBaseCode=PS  InternalSimscapePortConfiguration="{\"Bottom\":[],\"Left\":[{\"id\":\"DutyCycle\",\"label\":\"DutyCycle\",\"type\":\"input\"},{\"id\":\"p1\",\"label\":\"1+\",\"type\":\"foundation.electrical.electrical\"},{\"id\":\"n1\",\"label\":\"1-\",\"type\":\"foundation.electrical.electrical\"}],\"Right\":[{\"id\":\"p2\",\"label\":\"2+\",\"type\":\"foundation.electrical.electrical\"},{\"id\":\"n2\",\"label\":\"2-\",\"type\":\"foundation.electrical.electrical\"}],\"Top\":[]}"
  Current Sensor : fl_lib/Electrical/Electrical Sensors/Current Sensor
  Current Sensor (Three-Phase) : ee_lib/Sensors & Transducers/Current Sensor (Three-Phase)
  Electrical Reference1 : fl_lib/Electrical/Electrical Elements/Electrical Reference
  Line Voltage Sensor (Three-Phase) : ee_lib/Sensors & Transducers/Line Voltage Sensor (Three-Phase)
      settings: SourceProductBaseCode=PS
  PS-Simulink Converter{,1..3} (4 alike) : nesl_utility/PS-Simulink Converter  PhysicalDomain=network_engine_domain  SubClassName=ps_output  LeftPortType=input  RightPortType=output  PseudoPeriodic=off  Frequencies=[]  Unit=inherit  AffineConversion=off
  Product : Product
  Resistor : fl_lib/Electrical/Electrical Elements/Resistor  R=1e-5 Ohm  i_specify=off  i_priority=None  i=0 A  i_nominal_specify=off  i_nominal_unit=A  i_nominal_value=1  v_specify=off  v_priority=None  v=0 V  v_nominal_specify=off  v_nominal_unit=V  v_nominal_value=1
  Terminator : Terminator
  Terminator1 : Terminator
  Terminator2 : Terminator
  V2pu : Gain  Gain=1/12e3
  Voltage Source (Three-Phase) : ee_lib/Sources/Voltage Source (Three-Phase)  vline_rms=10e3 V  shift=0 deg  freq=60 Hz  impedance_option=2  SShortCircuit=1e6 V*A  XR=15  R=1e-5 Ohm  L=3.97e-4 H  G_parasitic=0 1/Ohm  harmonic_option=0  harmonic_orders=[5, 7, 11, 13]  harmonic_ratios=[.1, .1, .1, .1]  I_specify=off  I_priority=None  I=[ 0 0 0 ] A  I_nominal_specify=off  I_nominal_unit=A  I_nominal_value=1
      settings: SourceProductBaseCode=PS
  Voltage Sensor : fl_lib/Electrical/Electrical Sensors/Voltage Sensor
  breaker status : Subsystem
  breaker status Zone 1 : Subsystem
  droop : Gain  Gain=droop1
  voltage droop : Subsystem
  + : PMIOPort  Side=Right
  - : PMIOPort  Port=2  Side=Right
  wires:
  PS-Simulink Converter1/1 -> V2pu/1
  PS-Simulink Converter/1 -> A2pu/1
  breaker status Zone 1/1(status) -> breaker status/1(In1)
  A2pu/1 -> Product/2, droop/1  "IDC1"
  V2pu/1 -> Product/1, voltage droop/2(voltage)  "VDC1"
  Product/1 -> Terminator1/1  "PDC1"
  droop/1 -> voltage droop/1(droop)
  PS-Simulink Converter2/1 -> Terminator/1  "Iabc1"
  PS-Simulink Converter3/1 -> Terminator2/1  "Vabc1"
  connections:
  PS-Simulink Converter1/LConn1 -- Voltage Sensor/RConn1
  Voltage Sensor/RConn2 -- Average-Value DC-DC Converter/RConn2 -- -/RConn1
  Current Sensor/RConn2 -- Resistor/LConn1
  Current Sensor/RConn1 -- PS-Simulink Converter/LConn1
  Resistor/RConn1 -- Voltage Sensor/LConn1 -- +/RConn1
  Electrical Reference1/LConn1 -- Voltage Source (Three-Phase)/LConn1
  Average-Value Rectifier (Three-Phase)/RConn2 -- Average-Value DC-DC Converter/LConn3
  Average-Value DC-DC Converter/LConn2 -- Average-Value Rectifier (Three-Phase)/RConn1
  Average-Value DC-DC Converter/RConn1 -- Current Sensor/LConn1
  voltage droop/RConn1 -- Average-Value DC-DC Converter/LConn1
  PS-Simulink Converter3/LConn1 -- Line Voltage Sensor (Three-Phase)/RConn1
  Current Sensor (Three-Phase)/RConn1 -- PS-Simulink Converter2/LConn1
  Current Sensor (Three-Phase)/LConn1 -- Line Voltage Sensor (Three-Phase)/LConn1 -- Voltage Source (Three-Phase)/RConn1
  Current Sensor (Three-Phase)/RConn2 -- Average-Value Rectifier (Three-Phase)/LConn1

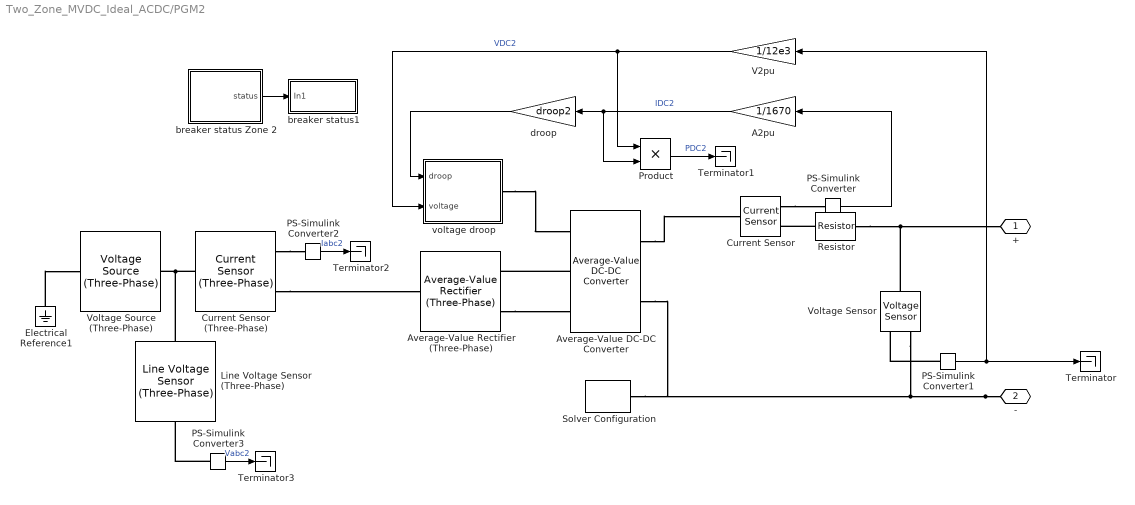
== system Two_Zone_MVDC_Ideal_ACDC/PGM2 ==
  A2pu : Gain  Gain=1/1670
  Average-Value Rectifier (Three-Phase) : ee_lib/Semiconductors & Converters/Converters/Average-Value Rectifier (Three-Phase)  VRated=12e3 V  Pfixed=1e4 W
      settings: SourceProductBaseCode=PS  InternalSimscapePortConfiguration="{\"Bottom\":[],\"Left\":[{\"id\":\"N\",\"label\":\"~\",\"type\":\"foundation.electrical.three_phase\"}],\"Right\":[{\"id\":\"p\",\"label\":\"+\",\"type\":\"foundation.electrical.electrical\"},{\"id\":\"n\",\"label\":\"-\",\"type\":\"foundation.electrical.electrical\"}],\"Top\":[]}"
  Average-Value DC-DC Converter : ee_lib/Semiconductors & Converters/Converters/Average-Value DC-DC Converter  control_option=ee.enum.converters.controlinput.dutycycle  converter_type=ee.enum.converters.dcdctype.buck  efficiency_option=ee.enum.converters.efficiency.constant  efficiency_fixed=100  i_vec=[0, 2, 5] A  efficiency_vec=[90, 95, 98]
      settings: SourceProductBaseCode=PS  InternalSimscapePortConfiguration="{\"Bottom\":[],\"Left\":[{\"id\":\"DutyCycle\",\"label\":\"DutyCycle\",\"type\":\"input\"},{\"id\":\"p1\",\"label\":\"1+\",\"type\":\"foundation.electrical.electrical\"},{\"id\":\"n1\",\"label\":\"1-\",\"type\":\"foundation.electrical.electrical\"}],\"Right\":[{\"id\":\"p2\",\"label\":\"2+\",\"type\":\"foundation.electrical.electrical\"},{\"id\":\"n2\",\"label\":\"2-\",\"type\":\"foundation.electrical.electrical\"}],\"Top\":[]}"
  Current Sensor : fl_lib/Electrical/Electrical Sensors/Current Sensor
  Current Sensor (Three-Phase) : ee_lib/Sensors & Transducers/Current Sensor (Three-Phase)
  Electrical Reference1 : fl_lib/Electrical/Electrical Elements/Electrical Reference
  Line Voltage Sensor (Three-Phase) : ee_lib/Sensors & Transducers/Line Voltage Sensor (Three-Phase)
      settings: SourceProductBaseCode=PS
  PS-Simulink Converter{,1..3} (4 alike) : nesl_utility/PS-Simulink Converter  PhysicalDomain=network_engine_domain  SubClassName=ps_output  LeftPortType=input  RightPortType=output  PseudoPeriodic=off  Frequencies=[]  Unit=inherit  AffineConversion=off
  Product : Product
  Resistor : fl_lib/Electrical/Electrical Elements/Resistor  R=1e-5 Ohm  i_specify=off  i_priority=None  i=0 A  i_nominal_specify=off  i_nominal_unit=A  i_nominal_value=1  v_specify=off  v_priority=None  v=0 V  v_nominal_specify=off  v_nominal_unit=V  v_nominal_value=1
  Solver Configuration : nesl_utility/Solver Configuration  PhysicalDomain=network_engine_domain  SubClassName=solver  LeftPortType=input  RightPortType=generic  Tones=[]  Harmonics=[]  SimulateNoise=off  Profile=off  UseLocalSampling=off  EnableSwitchedLinearOptims=on  FrequencyDomain=off  UseCCode=off  RelTol=0.001  AbsTol=1e-06  MinStep=1e-09  ToWorkspace=off  RevertToSquareIcSolve=off  NumHomotopyIterations=100  PhasorMode=off  PhasorModeNumHarmonics=1  DoDC=off  ResidualTolerance=1e-09  UseLocalSolver=on  LocalSolverChoice=NE_BACKWARD_EULER_ADVANCER  LocalSolverSampleTime=TsELEC  DoFixedCost=on  MaxNonlinIter=1  MaxModeIter=2  ComputeImpulses=off  ImpulseIterations=2  LinearAlgebra=auto  EquationFormulation=NE_TIME_EF  DelaysMemoryBudget=1024  AutomaticFiltering=on  FilteringTimeConstant=0.001  PartitionStorageMethod=AS_NEEDED  PartitionMemoryBudget=1024  PartitionMethod=FAST
  Terminator{,1..3} (4 alike) : Terminator
  V2pu : Gain  Gain=1/12e3
  Voltage Source (Three-Phase) : ee_lib/Sources/Voltage Source (Three-Phase)  vline_rms=10e3 V  shift=0 deg  freq=60 Hz  impedance_option=2  SShortCircuit=1e6 V*A  XR=15  R=1e-5 Ohm  L=3.97e-4 H  G_parasitic=0 1/Ohm  harmonic_option=0  harmonic_orders=[5, 7, 11, 13]  harmonic_ratios=[.1, .1, .1, .1]  I_specify=off  I_priority=None  I=[ 0 0 0 ] A  I_nominal_specify=off  I_nominal_unit=A  I_nominal_value=1
      settings: SourceProductBaseCode=PS
  Voltage Sensor : fl_lib/Electrical/Electrical Sensors/Voltage Sensor
  breaker status Zone 2 : Subsystem
  breaker status1 : Subsystem
  droop : Gain  Gain=droop2
  voltage droop : Subsystem
  + : PMIOPort  Side=Right
  - : PMIOPort  Port=2  Side=Right
  wires:
  PS-Simulink Converter/1 -> A2pu/1
  PS-Simulink Converter1/1 -> V2pu/1, Terminator/1
  breaker status Zone 2/1(status) -> breaker status1/1(In1)
  A2pu/1 -> Product/2, droop/1  "IDC2"
  Product/1 -> Terminator1/1  "PDC2"
  V2pu/1 -> Product/1, voltage droop/2(voltage)  "VDC2"
  droop/1 -> voltage droop/1(droop)
  PS-Simulink Converter3/1 -> Terminator3/1  "Vabc2"
  PS-Simulink Converter2/1 -> Terminator2/1  "Iabc2"
  connections:
  Resistor/RConn1 -- Voltage Sensor/LConn1 -- +/RConn1
  Current Sensor/RConn1 -- PS-Simulink Converter/LConn1
  Resistor/LConn1 -- Current Sensor/RConn2
  Average-Value DC-DC Converter/RConn1 -- Current Sensor/LConn1
  -/RConn1 -- Average-Value DC-DC Converter/RConn2 -- Solver Configuration/RConn1 -- Voltage Sensor/RConn2
  PS-Simulink Converter1/LConn1 -- Voltage Sensor/RConn1
  voltage droop/RConn1 -- Average-Value DC-DC Converter/LConn1
  Average-Value Rectifier (Three-Phase)/RConn2 -- Average-Value DC-DC Converter/LConn3
  Average-Value DC-DC Converter/LConn2 -- Average-Value Rectifier (Three-Phase)/RConn1
  Electrical Reference1/LConn1 -- Voltage Source (Three-Phase)/LConn1
  PS-Simulink Converter3/LConn1 -- Line Voltage Sensor (Three-Phase)/RConn1
  Current Sensor (Three-Phase)/RConn2 -- Average-Value Rectifier (Three-Phase)/LConn1
  Current Sensor (Three-Phase)/RConn1 -- PS-Simulink Converter2/LConn1
  Current Sensor (Three-Phase)/LConn1 -- Line Voltage Sensor (Three-Phase)/LConn1 -- Voltage Source (Three-Phase)/RConn1

== system Two_Zone_MVDC_Ideal_ACDC/SADA ==
  SADA : ee_lib/Switches & Breakers/DPST Switch  R_closed=1e-4 Ohm  G_open=1e-6 S  Threshold=0.5 V  Width=0 V  model_dynamics=0  t_on=1e-3 s  t_off=1e-3 s  initial_vT=0 V
      settings: SourceProductBaseCode=PS  InternalSimscapePortConfiguration="{\"Bottom\":[],\"Left\":[{\"id\":\"vT\",\"label\":\"vT\",\"type\":\"input\"},{\"id\":\"p1\",\"label\":\"\",\"type\":\"foundation.electrical.electrical\"},{\"id\":\"p2\",\"label\":\"\",\"type\":\"foundation.electrical.electrical\"}],\"Right\":[{\"id\":\"n1\",\"label\":\"\",\"type\":\"foundation.electrical.electrical\"},{\"id\":\"n2\",\"label\":\"\",\"type\":\"foundation.electrical.electrical\"}],\"Top\":[]}"
  Simulink-PS Converter : nesl_utility/Simulink-PS Converter  PhysicalDomain=network_engine_domain  SubClassName=ps_input  LeftPortType=input  RightPortType=output  PseudoPeriodic=off  Frequencies=[]  NoiseDistribution=none  NoiseParameters=[]  Unit=1  AffineConversion=off  FilteringAndDerivatives=provide  SimscapeFilterOrder=1  InputFilterTimeConstant=0.001  UdotUserProvided=0
  "+ " : PMIOPort  Side=Right
  + : PMIOPort  Port=2  Side=Left
  "- " : PMIOPort  Port=3  Side=Right
  - : PMIOPort  Port=4  Side=Left
  wires:
  [SADA] -> Simulink-PS Converter/1
  connections:
  SADA/RConn1 -- "+ "/RConn1
  SADA/LConn3 -- -/RConn1
  SADA/RConn2 -- "- "/RConn1
  Simulink-PS Converter/RConn1 -- SADA/LConn1
  SADA/LConn2 -- +/RConn1

== system Two_Zone_MVDC_Ideal_ACDC/SADB ==
  SADB : ee_lib/Switches & Breakers/DPST Switch  R_closed=1e-4 Ohm  G_open=1e-6 S  Threshold=0.5 V  Width=0 V  model_dynamics=0  t_on=1e-3 s  t_off=1e-3 s  initial_vT=0 V
      settings: SourceProductBaseCode=PS  InternalSimscapePortConfiguration="{\"Bottom\":[],\"Left\":[{\"id\":\"vT\",\"label\":\"vT\",\"type\":\"input\"},{\"id\":\"p1\",\"label\":\"\",\"type\":\"foundation.electrical.electrical\"},{\"id\":\"p2\",\"label\":\"\",\"type\":\"foundation.electrical.electrical\"}],\"Right\":[{\"id\":\"n1\",\"label\":\"\",\"type\":\"foundation.electrical.electrical\"},{\"id\":\"n2\",\"label\":\"\",\"type\":\"foundation.electrical.electrical\"}],\"Top\":[]}"
  Simulink-PS Converter : nesl_utility/Simulink-PS Converter  PhysicalDomain=network_engine_domain  SubClassName=ps_input  LeftPortType=input  RightPortType=output  PseudoPeriodic=off  Frequencies=[]  NoiseDistribution=none  NoiseParameters=[]  Unit=1  AffineConversion=off  FilteringAndDerivatives=provide  SimscapeFilterOrder=1  InputFilterTimeConstant=0.001  UdotUserProvided=0
  "+ " : PMIOPort  Side=Right
  + : PMIOPort  Port=2  Side=Left
  "- " : PMIOPort  Port=3  Side=Right
  - : PMIOPort  Port=4  Side=Left
  wires:
  [SADB] -> Simulink-PS Converter/1
  connections:
  SADB/LConn2 -- +/RConn1
  Simulink-PS Converter/RConn1 -- SADB/LConn1
  SADB/RConn2 -- "- "/RConn1
  SADB/LConn3 -- -/RConn1
  SADB/RConn1 -- "+ "/RConn1

== system Two_Zone_MVDC_Ideal_ACDC/SADC ==
  SADC : ee_lib/Switches & Breakers/DPST Switch  R_closed=1e-4 Ohm  G_open=1e-6 S  Threshold=0.5 V  Width=0 V  model_dynamics=0  t_on=1e-3 s  t_off=1e-3 s  initial_vT=0 V
      settings: SourceProductBaseCode=PS  InternalSimscapePortConfiguration="{\"Bottom\":[],\"Left\":[{\"id\":\"vT\",\"label\":\"vT\",\"type\":\"input\"},{\"id\":\"p1\",\"label\":\"\",\"type\":\"foundation.electrical.electrical\"},{\"id\":\"p2\",\"label\":\"\",\"type\":\"foundation.electrical.electrical\"}],\"Right\":[{\"id\":\"n1\",\"label\":\"\",\"type\":\"foundation.electrical.electrical\"},{\"id\":\"n2\",\"label\":\"\",\"type\":\"foundation.electrical.electrical\"}],\"Top\":[]}"
  Simulink-PS Converter : nesl_utility/Simulink-PS Converter  PhysicalDomain=network_engine_domain  SubClassName=ps_input  LeftPortType=input  RightPortType=output  PseudoPeriodic=off  Frequencies=[]  NoiseDistribution=none  NoiseParameters=[]  Unit=1  AffineConversion=off  FilteringAndDerivatives=provide  SimscapeFilterOrder=1  InputFilterTimeConstant=0.001  UdotUserProvided=0
  "+ " : PMIOPort  Side=Right
  + : PMIOPort  Port=2  Side=Left
  "- " : PMIOPort  Port=3  Side=Right
  - : PMIOPort  Port=4  Side=Left
  wires:
  [SADC] -> Simulink-PS Converter/1
  connections:
  SADC/LConn2 -- +/RConn1
  Simulink-PS Converter/RConn1 -- SADC/LConn1
  SADC/RConn2 -- "- "/RConn1
  SADC/LConn3 -- -/RConn1
  SADC/RConn1 -- "+ "/RConn1
